simulink model "Consigna5_2_1"  (R2024b)
settings: Solver=ode45  StartTime=0.0  StopTime=20  RelTol=1e-3
values from neighbouring files (symbols this model uses):
  A_corrientes = [0 1; -omega_n_corrientes^2 -2*omega_n_corrientes]    [parametros.m]
  A_inversor = [0 1; -omega_n_inversor^2 -2*omega_n_inversor]    [parametros.m]
  A_posicion = [0 1; -omega_n_posicion^2 -2*omega_n_posicion]    [parametros.m]
  A_temp = -1/20    (= -0.05)    [parametros.m]
  alpha_cu = 3.9 *10^-3    (= 0.0039)    [parametros.m]
  B_corrientes = [0; omega_n_corrientes^2]    [parametros.m]
  b_eq = b_m + (1/r^2) * b_l    (= 2.19444444444e-05)    [parametros.m]
  B_inversor = [0; omega_n_inversor^2]    [parametros.m]
  b_l = 0.1    [parametros.m]
  b_m = 1.5 * 10^-5    (= 1.5e-05)    [parametros.m]
  B_posicion = [0; omega_n_posicion^2]    [parametros.m]
  B_temp = 1/20    (= 0.05)    [parametros.m]
  ba = J_eq*n*omega_pos    (= 0.0916527777778)    [parametros.m]
  C_corrientes = [1 0]    [parametros.m]
  C_inversor = [1 0]    [parametros.m]
  C_posicion = [1 0]    [parametros.m]
  C_temp = 1    [parametros.m]
  C_ts = 0.818    [parametros.m]
  g = 9.80665    [parametros.m]
  J_l = (m*l_cm^2 + J_cm) + (m_l * l_l^2)    (= 0.4583)    [parametros.m]
  J_m = 1.4 * 10^-5    (= 1.4e-05)    [parametros.m]
  K_e_int = 3200 ^3    (= 32768000000)    [parametros.m]
  K_e_omega = 3*3200^2    (= 30720000)    [parametros.m]
  K_e_theta = 9600    [parametros.m]
  k_l = m * l_cm + m_l* l_l    (= 1)    [parametros.m]
  Ksa = J_eq*n*(omega_pos^2)    (= 73.3222222222)    [parametros.m]
  Ksia = J_eq*(omega_pos^3)    (= 23463.1111111)    [parametros.m]
  L_d = 6.6 * 10^-3    (= 0.0066)    [parametros.m]
  L_ls = 0.8 * 10^-3    (= 0.0008)    [parametros.m]
  L_q = 5.8 * 10^-3    (= 0.0058)    [parametros.m]
  lambda_m = 0.016    [parametros.m]
  P_p = 3    [parametros.m]
  r = 120    [parametros.m]
  R_s_40 = 1.02    [parametros.m]
  R_ts_amb = 146.7    [parametros.m]
  T_sample = 1/f_sample    (= 4.53514739229e-05)    [parametros.m]
  Temp_s_ref = 20    [parametros.m]
  tm = X(1)    [parametros.m]
  tr = X(2)    [parametros.m]
  w2 = 188.49556    [parametros.m]
  x0_corrientes = [0;0]    [parametros.m]
  x0_inversor = [0;0]    [parametros.m]
  x0_posicion = [0; 0]    [parametros.m]
  x0_temp = 20    [parametros.m]
libraries: simulink x14, dspsigops x6
(part 3 of 4)

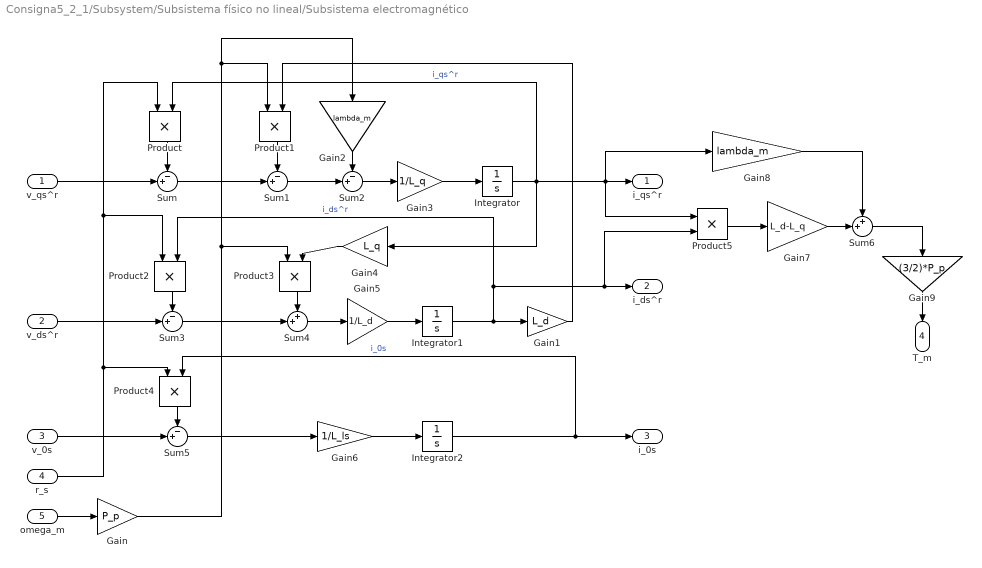
== system Consigna5_2_1/Subsystem/Subsistema físico no lineal/Subsistema electromagnético ==
  v_qs^r : Inport
  v_ds^r : Inport  Port=2
  v_0s : Inport  Port=3
  r_s : Inport  Port=4
  omega_m : Inport  Port=5
  Gain : Gain  Gain=P_p
  Gain1 : Gain  Gain=L_d
  Gain2 : Gain  Gain=lambda_m
  Gain3 : Gain  Gain=1/L_q
  Gain4 : Gain  Gain=L_q
  Gain5 : Gain  Gain=1/L_d
  Gain6 : Gain  Gain=1/L_ls
  Gain7 : Gain  Gain=L_d-L_q
  Gain8 : Gain  Gain=lambda_m
  Gain9 : Gain  Gain=(3/2)*P_p
  Integrator : Integrator
  Integrator1 : Integrator
  Integrator2 : Integrator
  Product{,1..5} (6 alike) : Product
  Sum{,1..3,5} (5 alike) : Sum  Inputs=-+|
  Sum4 : Sum  Inputs=++|
  Sum6 : Sum  Inputs=++|
  i_qs^r : Outport
  i_ds^r : Outport  Port=2
  i_0s : Outport  Port=3
  T_m : Outport  Port=4
  wires:
  v_qs^r/1 -> Sum/2
  Product/1 -> Sum/1
  Sum/1 -> Sum1/2
  Integrator/1 -> Gain8/1, Product5/1, i_qs^r/1, Product/2, Gain4/1  "i_qs^r"
  omega_m/1 -> Gain/1
  Gain/1 -> Gain2/1, Product1/1, Product3/1
  Integrator1/1 -> Product2/2, Product5/2, i_ds^r/1, Gain1/1  "i_ds^r"
  Gain1/1 -> Product1/2
  Sum1/1 -> Sum2/2
  Sum2/1 -> Gain3/1
  Gain2/1 -> Sum2/1
  Product1/1 -> Sum1/1
  Gain3/1 -> Integrator/1
  Product2/1 -> Sum3/1
  v_ds^r/1 -> Sum3/2
  Sum3/1 -> Sum4/2
  Product3/1 -> Sum4/1
  Gain4/1 -> Product3/2
  Gain5/1 -> Integrator1/1
  Sum4/1 -> Gain5/1
  Integrator2/1 -> Product4/2, i_0s/1  "i_0s"
  r_s/1 -> Product4/1, Product/1, Product2/1
  Product4/1 -> Sum5/1
  v_0s/1 -> Sum5/2
  Sum5/1 -> Gain6/1
  Gain6/1 -> Integrator2/1
  Product5/1 -> Gain7/1
  Gain7/1 -> Sum6/2
  Gain8/1 -> Sum6/1
  Sum6/1 -> Gain9/1
  Gain9/1 -> T_m/1

== system Consigna5_2_1/Subsystem/Subsistema físico no lineal/Subsistema mecánico completo ==
  T_m : Inport
  T_l : Inport  Port=2
  Gain : Gain  Gain=b_m + b_l / (r^2)
  Gain1 : Gain  Gain=1/r
  Gain2 : Gain  Gain=1/(J_m + J_l / r^2)
  Scope : Scope
  Sum : Sum  Inputs=-+-
  omega_m(0) = 0 : Integrator
  theta_m(0) = pi/4 : Integrator  InitialCondition=pi/4
  theta_m(t) : Outport
  omega_m(t) : Outport  Port=2
  wires:
  Gain2/1 -> omega_m(0) = 0/1  "domega_m(t)/dt"
  Gain1/1 -> Sum/1
  theta_m(0) = pi/4/1 -> Scope/1, theta_m(t)/1  "theta_m(t)"
  omega_m(0) = 0/1 -> omega_m(t)/1, Gain/1, theta_m(0) = pi/4/1  "omega_m(t)"
  Sum/1 -> Gain2/1
  Gain/1 -> Sum/3
  T_l/1 -> Gain1/1
  T_m/1 -> Sum/2

== system Consigna5_2_1/Subsystem/Subsistema físico no lineal/Subsistema térmico ==
  i_qs^r : Inport
  i_ds^r : Inport  Port=2
  i_0s^r : Inport  Port=3
  Tº_amb : Inport  Port=4
  Constant : Constant  Value=Temp_s_ref
  Constant1 : Constant
  Gain : Gain  Gain=1/C_ts
  Gain1 : Gain  Gain=3/2
  Gain2 : Gain  Gain=1/R_ts_amb
  Gain3 : Gain  Gain=alpha_cu
  Gain4 : Gain  Gain=R_s_40
  Gain5 : Gain  Gain=2
  Integrator : Integrator  InitialCondition=20
  Product : Product
  Square : Math  Operator=square
  Square1 : Math  Operator=square
  Square2 : Math  Operator=square
  Sum : Sum  Inputs=+++
  Sum1 : Sum  Inputs=-|+
  Sum2 : Sum  Inputs=|+-
  Sum3 : Sum  Inputs=|+-
  Sum4 : Sum  Inputs=|++
  r_s : Outport
  T_s : Outport  Port=2
  wires:
  i_qs^r/1 -> Square/1
  i_ds^r/1 -> Square1/1
  i_0s^r/1 -> Square2/1
  Gain/1 -> Integrator/1
  Square/1 -> Sum/1
  Square1/1 -> Sum/2
  Sum/1 -> Product/1
  Product/1 -> Gain1/1
  Tº_amb/1 -> Sum1/1
  Integrator/1 -> T_s/1, Sum3/1, Sum1/2
  Sum1/1 -> Gain2/1
  Gain1/1 -> Sum2/1
  Gain2/1 -> Sum2/2
  Sum2/1 -> Gain/1
  Constant/1 -> Sum3/2
  Sum3/1 -> Gain3/1
  Gain3/1 -> Sum4/1
  Constant1/1 -> Sum4/2
  Sum4/1 -> Gain4/1
  Gain4/1 -> Product/2, r_s/1
  Square2/1 -> Gain5/1
  Gain5/1 -> Sum/3

== system Consigna5_2_1/Subsystem/Subsystem2/Desacoples Fisicos ==
  v_qs* : Inport
  v_ds* : Inport  Port=2
  v_0s* : Inport  Port=3
  i_qs : Inport  Port=4
  i_ds : Inport  Port=5
  i_0s : Inport  Port=6
  omega_m : Inport  Port=7
  R_s : Inport  Port=8
  Constant : Constant  Value=lambda_m
  Gain : Gain  Gain=P_p
  Gain1 : Gain  Gain=L_d
  Gain2 : Gain  Gain=L_q*P_p
  Product{,1..4} (5 alike) : Product
  Sum : Sum  Inputs=|++
  Sum1 : Sum  Inputs=|++
  Sum2 : Sum  Inputs=++|
  Sum3 : Sum  Inputs=+-|
  Sum4 : Sum  Inputs=|++
  Sum5 : Sum  Inputs=++|
  v_qs*' : Outport
  v_ds*' : Outport  Port=2
  v_0s*' : Outport  Port=3
  wires:
  Gain/1 -> Product1/2
  Product2/1 -> Sum3/1
  Sum2/1 -> Product1/1
  Sum1/1 -> v_qs*'/1
  i_ds/1 -> Gain1/1, Product2/2
  i_qs/1 -> Gain2/1, Product/2
  v_qs*/1 -> Sum/1
  v_0s*/1 -> Sum5/2
  v_ds*/1 -> Sum4/1
  Sum/1 -> Sum1/1
  R_s/1 -> Product2/1, Product4/1, Product/1
  Sum4/1 -> v_ds*'/1
  Gain2/1 -> Product3/1
  Sum5/1 -> v_0s*'/1
  Product3/1 -> Sum3/2
  omega_m/1 -> Product3/2, Gain/1
  Constant/1 -> Sum2/1
  Product/1 -> Sum/2
  Gain1/1 -> Sum2/2
  Sum3/1 -> Sum4/2
  Product4/1 -> Sum5/1
  i_0s/1 -> Product4/2
  Product1/1 -> Sum1/2

== system Consigna5_2_1/Subsystem/Subsystem2/Lazo de Torque ==
  Tm* : Inport
  omega_m : Inport  Port=2
  ids : Inport  Port=3
  Constant : Constant  Value=lambda_m
  Constant1 : Constant  Value=g
  Divide : Product  Inputs=*/
  Integrator : Integrator  InitialCondition=pi/4
  Ld-Lq : Constant  Value=L_d-L_q
  Multiply : Gain  Gain=b_eq
  Multiply1 : Gain  Gain=1/r
  Multiply2 : Gain  Gain=k_l
  Multiply3 : Gain  Gain=1/r
  Multiply5 : Gain  Gain=P_p
  Multiply6 : Gain  Gain=3/2
  Product : Product
  Product1 : Product
  Sin : Trigonometry
  Sum1 : Sum  Inputs=|++
  Sum2 : Sum  Inputs=|+++
  iqs* : Outport
  wires:
  Constant/1 -> Sum1/2
  Ld-Lq/1 -> Product1/2
  omega_m/1 -> Integrator/1, Multiply/1
  Tm*/1 -> Sum2/1
  ids/1 -> Product1/1
  Multiply3/1 -> Product/1
  Product/1 -> Sum2/3
  Multiply6/1 -> Divide/2
  Multiply2/1 -> Multiply3/1
  Integrator/1 -> Multiply1/1
  Multiply1/1 -> Sin/1
  Multiply/1 -> Sum2/2
  Sum2/1 -> Divide/1
  Multiply5/1 -> Multiply6/1
  Divide/1 -> iqs*/1
  Sum1/1 -> Multiply5/1
  Sin/1 -> Multiply2/1
  Constant1/1 -> Product/2
  Product1/1 -> Sum1/1

== system Consigna5_2_1/Subsystem/Subsystem2/Modulador de corriente ==
  I_qs* : Inport
  I_ds* : Inport  Port=2
  I_0s* : Inport  Port=3
  i_qs : Inport  Port=4
  i_ds : Inport  Port=5
  i_0s : Inport  Port=6
  Gain : Gain  Gain=5000*L_q
  Gain1 : Gain  Gain=5000*L_d
  Gain2 : Gain  Gain=5000*L_ls
  Sum : Sum  Inputs=+-
  Sum1 : Sum  Inputs=+-
  Sum2 : Sum  Inputs=+-
  v_qs* : Outport
  v_ds* : Outport  Port=2
  v_0s* : Outport  Port=3
  wires:
  Sum2/1 -> Gain2/1
  Sum1/1 -> Gain1/1
  Sum/1 -> Gain/1
  I_qs*/1 -> Sum/1
  i_qs/1 -> Sum/2
  I_ds*/1 -> Sum1/1
  i_ds/1 -> Sum1/2
  I_0s*/1 -> Sum2/1
  i_0s/1 -> Sum2/2
  Gain/1 -> v_qs*/1
  Gain2/1 -> v_0s*/1
  Gain1/1 -> v_ds*/1

== system Consigna5_2_1/Subsystem1/MODULADOR DE TORQUE1/Calculo rs ==
  Ts : Inport
  Constant : Constant
  Constant1 : Constant  Value=Temp_s_ref
  Gain : Gain  Gain=alpha_cu
  Gain1 : Gain  Gain=R_s_40
  Sum : Sum  Inputs=|++
  Sum1 : Sum  Inputs=|-+
  r_s : Outport
  wires:
  Constant/1 -> Sum/1
  Gain/1 -> Sum/2
  Ts/1 -> Sum1/2
  Constant1/1 -> Sum1/1
  Sum1/1 -> Gain/1
  Sum/1 -> Gain1/1
  Gain1/1 -> r_s/1

== system Consigna5_2_1/Subsystem1/MODULADOR DE TORQUE1/Desacoples Fisicos ==
  v_qs* : Inport
  v_ds* : Inport  Port=2
  v_0s* : Inport  Port=3
  i_qs : Inport  Port=4
  i_ds : Inport  Port=5
  i_0s : Inport  Port=6
  omega_m : Inport  Port=7
  R_s : Inport  Port=8
  Constant : Constant  Value=lambda_m
  Gain : Gain  Gain=P_p
  Gain1 : Gain  Gain=L_d
  Gain2 : Gain  Gain=L_q*P_p
  Product{,1..4} (5 alike) : Product
  Sum : Sum  Inputs=|++
  Sum1 : Sum  Inputs=|++
  Sum2 : Sum  Inputs=++|
  Sum3 : Sum  Inputs=+-|
  Sum4 : Sum  Inputs=|++
  Sum5 : Sum  Inputs=++|
  v_qs*' : Outport
  v_ds*' : Outport  Port=2
  v_0s*' : Outport  Port=3
  wires:
  Gain/1 -> Product1/2
  Product2/1 -> Sum3/1
  Sum2/1 -> Product1/1
  Sum1/1 -> v_qs*'/1
  i_ds/1 -> Gain1/1, Product2/2
  i_qs/1 -> Gain2/1, Product/2
  v_qs*/1 -> Sum/1
  v_0s*/1 -> Sum5/2
  v_ds*/1 -> Sum4/1
  Sum/1 -> Sum1/1
  R_s/1 -> Product2/1, Product4/1, Product/1
  Sum4/1 -> v_ds*'/1
  Gain2/1 -> Product3/1
  Sum5/1 -> v_0s*'/1
  Product3/1 -> Sum3/2
  omega_m/1 -> Product3/2, Gain/1
  Constant/1 -> Sum2/1
  Product/1 -> Sum/2
  Gain1/1 -> Sum2/2
  Sum3/1 -> Sum4/2
  Product4/1 -> Sum5/1
  i_0s/1 -> Product4/2
  Product1/1 -> Sum1/2

== system Consigna5_2_1/Subsystem1/MODULADOR DE TORQUE1/Lazo de Torque ==
  Tm* : Inport
  omega_m : Inport  Port=2
  ids : Inport  Port=3
  Constant : Constant  Value=lambda_m
  Constant1 : Constant  Value=g
  Divide : Product  Inputs=*/
  Integrator : Integrator  InitialCondition=pi/4
  Ld-Lq : Constant  Value=L_d-L_q
  Multiply : Gain  Gain=b_eq
  Multiply1 : Gain  Gain=1/r
  Multiply2 : Gain  Gain=k_l
  Multiply3 : Gain  Gain=1/r
  Multiply5 : Gain  Gain=P_p
  Multiply6 : Gain  Gain=3/2
  Product : Product
  Product1 : Product
  Sin : Trigonometry
  Sum1 : Sum  Inputs=|++
  Sum2 : Sum  Inputs=|+++
  iqs* : Outport
  wires:
  Constant/1 -> Sum1/2
  Ld-Lq/1 -> Product1/2
  omega_m/1 -> Integrator/1, Multiply/1
  Tm*/1 -> Sum2/1
  ids/1 -> Product1/1
  Multiply3/1 -> Product/1
  Product/1 -> Sum2/3
  Multiply6/1 -> Divide/2
  Multiply2/1 -> Multiply3/1
  Integrator/1 -> Multiply1/1
  Multiply1/1 -> Sin/1
  Multiply/1 -> Sum2/2
  Sum2/1 -> Divide/1
  Multiply5/1 -> Multiply6/1
  Divide/1 -> iqs*/1
  Sum1/1 -> Multiply5/1
  Sin/1 -> Multiply2/1
  Constant1/1 -> Product/2
  Product1/1 -> Sum1/1

== system Consigna5_2_1/Subsystem1/MODULADOR DE TORQUE1/Modulador de corriente ==
  I_qs* : Inport
  I_ds* : Inport  Port=2
  I_0s* : Inport  Port=3
  i_qs : Inport  Port=4
  i_ds : Inport  Port=5
  i_0s : Inport  Port=6
  Gain : Gain  Gain=5000*L_q
  Gain1 : Gain  Gain=5000*L_d
  Gain2 : Gain  Gain=5000*L_ls
  Sum : Sum  Inputs=+-
  Sum1 : Sum  Inputs=+-
  Sum2 : Sum  Inputs=+-
  v_qs* : Outport
  v_ds* : Outport  Port=2
  v_0s* : Outport  Port=3
  wires:
  Sum2/1 -> Gain2/1
  Sum1/1 -> Gain1/1
  Sum/1 -> Gain/1
  I_qs*/1 -> Sum/1
  i_qs/1 -> Sum/2
  I_ds*/1 -> Sum1/1
  i_ds/1 -> Sum1/2
  I_0s*/1 -> Sum2/1
  i_0s/1 -> Sum2/2
  Gain/1 -> v_qs*/1
  Gain2/1 -> v_0s*/1
  Gain1/1 -> v_ds*/1

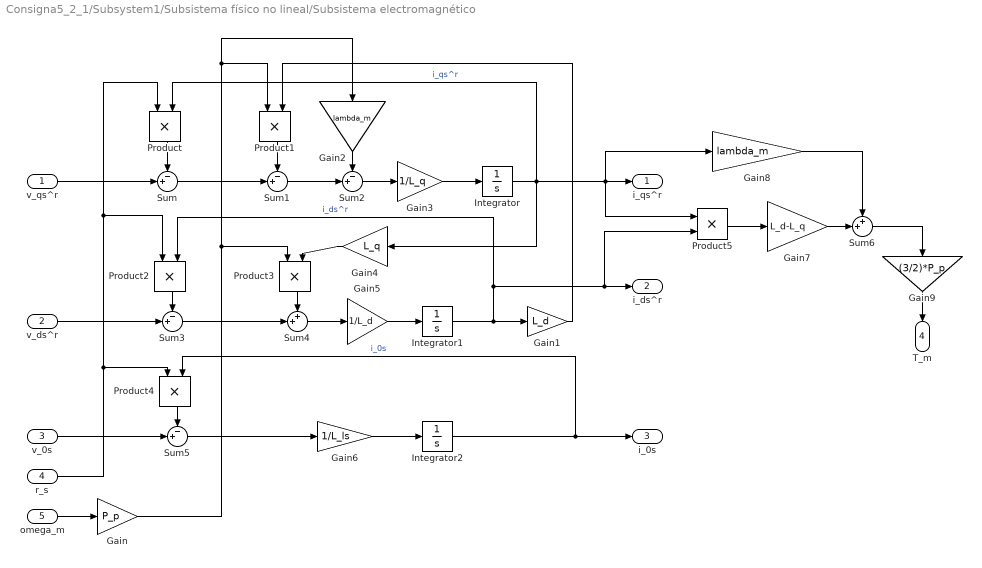
== system Consigna5_2_1/Subsystem1/Subsistema físico no lineal/Subsistema electromagnético ==
  v_qs^r : Inport
  v_ds^r : Inport  Port=2
  v_0s : Inport  Port=3
  r_s : Inport  Port=4
  omega_m : Inport  Port=5
  Gain : Gain  Gain=P_p
  Gain1 : Gain  Gain=L_d
  Gain2 : Gain  Gain=lambda_m
  Gain3 : Gain  Gain=1/L_q
  Gain4 : Gain  Gain=L_q
  Gain5 : Gain  Gain=1/L_d
  Gain6 : Gain  Gain=1/L_ls
  Gain7 : Gain  Gain=L_d-L_q
  Gain8 : Gain  Gain=lambda_m
  Gain9 : Gain  Gain=(3/2)*P_p
  Integrator : Integrator
  Integrator1 : Integrator
  Integrator2 : Integrator
  Product{,1..5} (6 alike) : Product
  Sum{,1..3,5} (5 alike) : Sum  Inputs=-+|
  Sum4 : Sum  Inputs=++|
  Sum6 : Sum  Inputs=++|
  i_qs^r : Outport
  i_ds^r : Outport  Port=2
  i_0s : Outport  Port=3
  T_m : Outport  Port=4
  wires:
  v_qs^r/1 -> Sum/2
  Product/1 -> Sum/1
  Sum/1 -> Sum1/2
  Integrator/1 -> Gain8/1, Product5/1, i_qs^r/1, Product/2, Gain4/1  "i_qs^r"
  omega_m/1 -> Gain/1
  Gain/1 -> Gain2/1, Product1/1, Product3/1
  Integrator1/1 -> Product2/2, Product5/2, i_ds^r/1, Gain1/1  "i_ds^r"
  Gain1/1 -> Product1/2
  Sum1/1 -> Sum2/2
  Sum2/1 -> Gain3/1
  Gain2/1 -> Sum2/1
  Product1/1 -> Sum1/1
  Gain3/1 -> Integrator/1
  Product2/1 -> Sum3/1
  v_ds^r/1 -> Sum3/2
  Sum3/1 -> Sum4/2
  Product3/1 -> Sum4/1
  Gain4/1 -> Product3/2
  Gain5/1 -> Integrator1/1
  Sum4/1 -> Gain5/1
  Integrator2/1 -> Product4/2, i_0s/1  "i_0s"
  r_s/1 -> Product4/1, Product/1, Product2/1
  Product4/1 -> Sum5/1
  v_0s/1 -> Sum5/2
  Sum5/1 -> Gain6/1
  Gain6/1 -> Integrator2/1
  Product5/1 -> Gain7/1
  Gain7/1 -> Sum6/2
  Gain8/1 -> Sum6/1
  Sum6/1 -> Gain9/1
  Gain9/1 -> T_m/1

== system Consigna5_2_1/Subsystem1/Subsistema físico no lineal/Subsistema mecánico completo ==
  T_m : Inport
  T_l : Inport  Port=2
  Gain : Gain  Gain=b_m + b_l / (r^2)
  Gain1 : Gain  Gain=1/r
  Gain2 : Gain  Gain=1/(J_m + J_l / r^2)
  Sum : Sum  Inputs=-+-
  omega_m(0) = 0 : Integrator
  theta_m(0) = 0 : Integrator
  theta_m(t) : Outport
  omega_m(t) : Outport  Port=2
  wires:
  Gain2/1 -> omega_m(0) = 0/1  "domega_m(t)/dt"
  Gain1/1 -> Sum/1
  theta_m(0) = 0/1 -> theta_m(t)/1  "theta_m(t)"
  omega_m(0) = 0/1 -> omega_m(t)/1, Gain/1, theta_m(0) = 0/1  "omega_m(t)"
  Sum/1 -> Gain2/1
  Gain/1 -> Sum/3
  T_l/1 -> Gain1/1
  T_m/1 -> Sum/2

== system Consigna5_2_1/Subsystem1/Subsistema físico no lineal/Subsistema térmico ==
  i_qs^r : Inport
  i_ds^r : Inport  Port=2
  i_0s^r : Inport  Port=3
  Tº_amb : Inport  Port=4
  Constant : Constant  Value=Temp_s_ref
  Constant1 : Constant
  Gain : Gain  Gain=1/C_ts
  Gain1 : Gain  Gain=3/2
  Gain2 : Gain  Gain=1/R_ts_amb
  Gain3 : Gain  Gain=alpha_cu
  Gain4 : Gain  Gain=R_s_40
  Gain5 : Gain  Gain=2
  Integrator : Integrator  InitialCondition=20
  Product : Product
  Square : Math  Operator=square
  Square1 : Math  Operator=square
  Square2 : Math  Operator=square
  Sum : Sum  Inputs=+++
  Sum1 : Sum  Inputs=-|+
  Sum2 : Sum  Inputs=|+-
  Sum3 : Sum  Inputs=|+-
  Sum4 : Sum  Inputs=|++
  r_s : Outport
  T_s : Outport  Port=2
  wires:
  i_qs^r/1 -> Square/1
  i_ds^r/1 -> Square1/1
  i_0s^r/1 -> Square2/1
  Gain/1 -> Integrator/1
  Square/1 -> Sum/1
  Square1/1 -> Sum/2
  Sum/1 -> Product/1
  Product/1 -> Gain1/1
  Tº_amb/1 -> Sum1/1
  Integrator/1 -> T_s/1, Sum3/1, Sum1/2
  Sum1/1 -> Gain2/1
  Gain1/1 -> Sum2/1
  Gain2/1 -> Sum2/2
  Sum2/1 -> Gain/1
  Constant/1 -> Sum3/2
  Sum3/1 -> Gain3/1
  Gain3/1 -> Sum4/1
  Constant1/1 -> Sum4/2
  Sum4/1 -> Gain4/1
  Gain4/1 -> Product/2, r_s/1
  Square2/1 -> Gain5/1
  Gain5/1 -> Sum/3

== system Consigna5_2_1/Subsystem2/MODULADOR DE TORQUE1/Calculo rs ==
  Ts : Inport
  Constant : Constant
  Constant1 : Constant  Value=Temp_s_ref
  Gain : Gain  Gain=alpha_cu
  Gain1 : Gain  Gain=R_s_40
  Sum : Sum  Inputs=|++
  Sum1 : Sum  Inputs=|-+
  r_s : Outport
  wires:
  Constant/1 -> Sum/1
  Gain/1 -> Sum/2
  Ts/1 -> Sum1/2
  Constant1/1 -> Sum1/1
  Sum1/1 -> Gain/1
  Sum/1 -> Gain1/1
  Gain1/1 -> r_s/1

== system Consigna5_2_1/Subsystem2/MODULADOR DE TORQUE1/Desacoples Fisicos ==
  v_qs* : Inport
  v_ds* : Inport  Port=2
  v_0s* : Inport  Port=3
  i_qs : Inport  Port=4
  i_ds : Inport  Port=5
  i_0s : Inport  Port=6
  omega_m : Inport  Port=7
  R_s : Inport  Port=8
  Constant : Constant  Value=lambda_m
  Gain : Gain  Gain=P_p
  Gain1 : Gain  Gain=L_d
  Gain2 : Gain  Gain=L_q*P_p
  Product{,1..4} (5 alike) : Product
  Sum : Sum  Inputs=|++
  Sum1 : Sum  Inputs=|++
  Sum2 : Sum  Inputs=++|
  Sum3 : Sum  Inputs=+-|
  Sum4 : Sum  Inputs=|++
  Sum5 : Sum  Inputs=++|
  v_qs*' : Outport
  v_ds*' : Outport  Port=2
  v_0s*' : Outport  Port=3
  wires:
  Gain/1 -> Product1/2
  Product2/1 -> Sum3/1
  Sum2/1 -> Product1/1
  Sum1/1 -> v_qs*'/1
  i_ds/1 -> Gain1/1, Product2/2
  i_qs/1 -> Gain2/1, Product/2
  v_qs*/1 -> Sum/1
  v_0s*/1 -> Sum5/2
  v_ds*/1 -> Sum4/1
  Sum/1 -> Sum1/1
  R_s/1 -> Product2/1, Product4/1, Product/1
  Sum4/1 -> v_ds*'/1
  Gain2/1 -> Product3/1
  Sum5/1 -> v_0s*'/1
  Product3/1 -> Sum3/2
  omega_m/1 -> Product3/2, Gain/1
  Constant/1 -> Sum2/1
  Product/1 -> Sum/2
  Gain1/1 -> Sum2/2
  Sum3/1 -> Sum4/2
  Product4/1 -> Sum5/1
  i_0s/1 -> Product4/2
  Product1/1 -> Sum1/2

== system Consigna5_2_1/Subsystem2/MODULADOR DE TORQUE1/Lazo de Torque ==
  Tm* : Inport
  omega_m : Inport  Port=2
  ids : Inport  Port=3
  Constant : Constant  Value=lambda_m
  Constant1 : Constant  Value=g
  Divide : Product  Inputs=*/
  Integrator : Integrator  InitialCondition=pi/4
  Ld-Lq : Constant  Value=L_d-L_q
  Multiply : Gain  Gain=b_eq
  Multiply1 : Gain  Gain=1/r
  Multiply2 : Gain  Gain=k_l
  Multiply3 : Gain  Gain=1/r
  Multiply5 : Gain  Gain=P_p
  Multiply6 : Gain  Gain=3/2
  Product : Product
  Product1 : Product
  Sin : Trigonometry
  Sum1 : Sum  Inputs=|++
  Sum2 : Sum  Inputs=|+++
  iqs* : Outport
  wires:
  Constant/1 -> Sum1/2
  Ld-Lq/1 -> Product1/2
  omega_m/1 -> Integrator/1, Multiply/1
  Tm*/1 -> Sum2/1
  ids/1 -> Product1/1
  Multiply3/1 -> Product/1
  Product/1 -> Sum2/3
  Multiply6/1 -> Divide/2
  Multiply2/1 -> Multiply3/1
  Integrator/1 -> Multiply1/1
  Multiply1/1 -> Sin/1
  Multiply/1 -> Sum2/2
  Sum2/1 -> Divide/1
  Multiply5/1 -> Multiply6/1
  Divide/1 -> iqs*/1
  Sum1/1 -> Multiply5/1
  Sin/1 -> Multiply2/1
  Constant1/1 -> Product/2
  Product1/1 -> Sum1/1

== system Consigna5_2_1/Subsystem2/MODULADOR DE TORQUE1/Modulador de corriente ==
  I_qs* : Inport
  I_ds* : Inport  Port=2
  I_0s* : Inport  Port=3
  i_qs : Inport  Port=4
  i_ds : Inport  Port=5
  i_0s : Inport  Port=6
  Gain : Gain  Gain=5000*L_q
  Gain1 : Gain  Gain=5000*L_d
  Gain2 : Gain  Gain=5000*L_ls
  Sum : Sum  Inputs=+-
  Sum1 : Sum  Inputs=+-
  Sum2 : Sum  Inputs=+-
  v_qs* : Outport
  v_ds* : Outport  Port=2
  v_0s* : Outport  Port=3
  wires:
  Sum2/1 -> Gain2/1
  Sum1/1 -> Gain1/1
  Sum/1 -> Gain/1
  I_qs*/1 -> Sum/1
  i_qs/1 -> Sum/2
  I_ds*/1 -> Sum1/1
  i_ds/1 -> Sum1/2
  I_0s*/1 -> Sum2/1
  i_0s/1 -> Sum2/2
  Gain/1 -> v_qs*/1
  Gain2/1 -> v_0s*/1
  Gain1/1 -> v_ds*/1

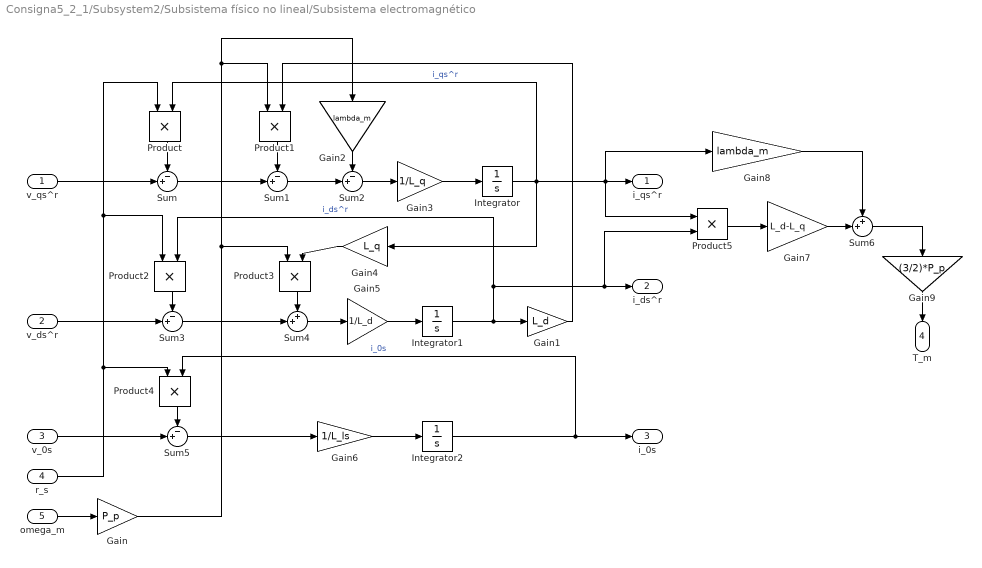
== system Consigna5_2_1/Subsystem2/Subsistema físico no lineal/Subsistema electromagnético ==
  v_qs^r : Inport
  v_ds^r : Inport  Port=2
  v_0s : Inport  Port=3
  r_s : Inport  Port=4
  omega_m : Inport  Port=5
  Gain : Gain  Gain=P_p
  Gain1 : Gain  Gain=L_d
  Gain2 : Gain  Gain=lambda_m
  Gain3 : Gain  Gain=1/L_q
  Gain4 : Gain  Gain=L_q
  Gain5 : Gain  Gain=1/L_d
  Gain6 : Gain  Gain=1/L_ls
  Gain7 : Gain  Gain=L_d-L_q
  Gain8 : Gain  Gain=lambda_m
  Gain9 : Gain  Gain=(3/2)*P_p
  Integrator : Integrator
  Integrator1 : Integrator
  Integrator2 : Integrator
  Product{,1..5} (6 alike) : Product
  Sum{,1..3,5} (5 alike) : Sum  Inputs=-+|
  Sum4 : Sum  Inputs=++|
  Sum6 : Sum  Inputs=++|
  i_qs^r : Outport
  i_ds^r : Outport  Port=2
  i_0s : Outport  Port=3
  T_m : Outport  Port=4
  wires:
  v_qs^r/1 -> Sum/2
  Product/1 -> Sum/1
  Sum/1 -> Sum1/2
  Integrator/1 -> Gain8/1, Product5/1, i_qs^r/1, Product/2, Gain4/1  "i_qs^r"
  omega_m/1 -> Gain/1
  Gain/1 -> Gain2/1, Product1/1, Product3/1
  Integrator1/1 -> Product2/2, Product5/2, i_ds^r/1, Gain1/1  "i_ds^r"
  Gain1/1 -> Product1/2
  Sum1/1 -> Sum2/2
  Sum2/1 -> Gain3/1
  Gain2/1 -> Sum2/1
  Product1/1 -> Sum1/1
  Gain3/1 -> Integrator/1
  Product2/1 -> Sum3/1
  v_ds^r/1 -> Sum3/2
  Sum3/1 -> Sum4/2
  Product3/1 -> Sum4/1
  Gain4/1 -> Product3/2
  Gain5/1 -> Integrator1/1
  Sum4/1 -> Gain5/1
  Integrator2/1 -> Product4/2, i_0s/1  "i_0s"
  r_s/1 -> Product4/1, Product/1, Product2/1
  Product4/1 -> Sum5/1
  v_0s/1 -> Sum5/2
  Sum5/1 -> Gain6/1
  Gain6/1 -> Integrator2/1
  Product5/1 -> Gain7/1
  Gain7/1 -> Sum6/2
  Gain8/1 -> Sum6/1
  Sum6/1 -> Gain9/1
  Gain9/1 -> T_m/1

== system Consigna5_2_1/Subsystem2/Subsistema físico no lineal/Subsistema mecánico completo ==
  T_m : Inport
  T_l : Inport  Port=2
  Gain : Gain  Gain=b_m + b_l / (r^2)
  Gain1 : Gain  Gain=1/r
  Gain2 : Gain  Gain=1/(J_m + J_l / r^2)
  Sum : Sum  Inputs=-+-
  omega_m(0) = 0 : Integrator
  theta_m(0) = 0 : Integrator
  theta_m(t) : Outport
  omega_m(t) : Outport  Port=2
  wires:
  Gain2/1 -> omega_m(0) = 0/1  "domega_m(t)/dt"
  Gain1/1 -> Sum/1
  theta_m(0) = 0/1 -> theta_m(t)/1  "theta_m(t)"
  omega_m(0) = 0/1 -> omega_m(t)/1, Gain/1, theta_m(0) = 0/1  "omega_m(t)"
  Sum/1 -> Gain2/1
  Gain/1 -> Sum/3
  T_l/1 -> Gain1/1
  T_m/1 -> Sum/2

== system Consigna5_2_1/Subsystem2/Subsistema físico no lineal/Subsistema térmico ==
  i_qs^r : Inport
  i_ds^r : Inport  Port=2
  i_0s^r : Inport  Port=3
  Tº_amb : Inport  Port=4
  Constant : Constant  Value=Temp_s_ref
  Constant1 : Constant
  Gain : Gain  Gain=1/C_ts
  Gain1 : Gain  Gain=3/2
  Gain2 : Gain  Gain=1/R_ts_amb
  Gain3 : Gain  Gain=alpha_cu
  Gain4 : Gain  Gain=R_s_40
  Gain5 : Gain  Gain=2
  Integrator : Integrator  InitialCondition=20
  Product : Product
  Square : Math  Operator=square
  Square1 : Math  Operator=square
  Square2 : Math  Operator=square
  Sum : Sum  Inputs=+++
  Sum1 : Sum  Inputs=-|+
  Sum2 : Sum  Inputs=|+-
  Sum3 : Sum  Inputs=|+-
  Sum4 : Sum  Inputs=|++
  r_s : Outport
  T_s : Outport  Port=2
  wires:
  i_qs^r/1 -> Square/1
  i_ds^r/1 -> Square1/1
  i_0s^r/1 -> Square2/1
  Gain/1 -> Integrator/1
  Square/1 -> Sum/1
  Square1/1 -> Sum/2
  Sum/1 -> Product/1
  Product/1 -> Gain1/1
  Tº_amb/1 -> Sum1/1
  Integrator/1 -> T_s/1, Sum3/1, Sum1/2
  Sum1/1 -> Gain2/1
  Gain1/1 -> Sum2/1
  Gain2/1 -> Sum2/2
  Sum2/1 -> Gain/1
  Constant/1 -> Sum3/2
  Sum3/1 -> Gain3/1
  Gain3/1 -> Sum4/1
  Constant1/1 -> Sum4/2
  Sum4/1 -> Gain4/1
  Gain4/1 -> Product/2, r_s/1
  Square2/1 -> Gain5/1
  Gain5/1 -> Sum/3

== system Consigna5_2_1/Subsystem3/MODULADOR DE TORQUE1/Calculo rs ==
  Ts : Inport
  Constant : Constant
  Constant1 : Constant  Value=Temp_s_ref
  Gain : Gain  Gain=alpha_cu
  Gain1 : Gain  Gain=R_s_40
  Sum : Sum  Inputs=|++
  Sum1 : Sum  Inputs=|-+
  r_s : Outport
  wires:
  Constant/1 -> Sum/1
  Gain/1 -> Sum/2
  Ts/1 -> Sum1/2
  Constant1/1 -> Sum1/1
  Sum1/1 -> Gain/1
  Sum/1 -> Gain1/1
  Gain1/1 -> r_s/1

== system Consigna5_2_1/Subsystem3/MODULADOR DE TORQUE1/Desacoples Fisicos ==
  v_qs* : Inport
  v_ds* : Inport  Port=2
  v_0s* : Inport  Port=3
  i_qs : Inport  Port=4
  i_ds : Inport  Port=5
  i_0s : Inport  Port=6
  omega_m : Inport  Port=7
  R_s : Inport  Port=8
  Constant : Constant  Value=lambda_m
  Gain : Gain  Gain=P_p
  Gain1 : Gain  Gain=L_d
  Gain2 : Gain  Gain=L_q*P_p
  Product{,1..4} (5 alike) : Product
  Sum : Sum  Inputs=|++
  Sum1 : Sum  Inputs=|++
  Sum2 : Sum  Inputs=++|
  Sum3 : Sum  Inputs=+-|
  Sum4 : Sum  Inputs=|++
  Sum5 : Sum  Inputs=++|
  v_qs*' : Outport
  v_ds*' : Outport  Port=2
  v_0s*' : Outport  Port=3
  wires:
  Gain/1 -> Product1/2
  Product2/1 -> Sum3/1
  Sum2/1 -> Product1/1
  Sum1/1 -> v_qs*'/1
  i_ds/1 -> Gain1/1, Product2/2
  i_qs/1 -> Gain2/1, Product/2
  v_qs*/1 -> Sum/1
  v_0s*/1 -> Sum5/2
  v_ds*/1 -> Sum4/1
  Sum/1 -> Sum1/1
  R_s/1 -> Product2/1, Product4/1, Product/1
  Sum4/1 -> v_ds*'/1
  Gain2/1 -> Product3/1
  Sum5/1 -> v_0s*'/1
  Product3/1 -> Sum3/2
  omega_m/1 -> Product3/2, Gain/1
  Constant/1 -> Sum2/1
  Product/1 -> Sum/2
  Gain1/1 -> Sum2/2
  Sum3/1 -> Sum4/2
  Product4/1 -> Sum5/1
  i_0s/1 -> Product4/2
  Product1/1 -> Sum1/2

== system Consigna5_2_1/Subsystem3/MODULADOR DE TORQUE1/Lazo de Torque ==
  Tm* : Inport
  omega_m : Inport  Port=2
  ids : Inport  Port=3
  Constant : Constant  Value=lambda_m
  Constant1 : Constant  Value=g
  Divide : Product  Inputs=*/
  Integrator : Integrator  InitialCondition=pi/4
  Ld-Lq : Constant  Value=L_d-L_q
  Multiply : Gain  Gain=b_eq
  Multiply1 : Gain  Gain=1/r
  Multiply2 : Gain  Gain=k_l
  Multiply3 : Gain  Gain=1/r
  Multiply5 : Gain  Gain=P_p
  Multiply6 : Gain  Gain=3/2
  Product : Product
  Product1 : Product
  Sin : Trigonometry
  Sum1 : Sum  Inputs=|++
  Sum2 : Sum  Inputs=|+++
  iqs* : Outport
  wires:
  Constant/1 -> Sum1/2
  Ld-Lq/1 -> Product1/2
  omega_m/1 -> Integrator/1, Multiply/1
  Tm*/1 -> Sum2/1
  ids/1 -> Product1/1
  Multiply3/1 -> Product/1
  Product/1 -> Sum2/3
  Multiply6/1 -> Divide/2
  Multiply2/1 -> Multiply3/1
  Integrator/1 -> Multiply1/1
  Multiply1/1 -> Sin/1
  Multiply/1 -> Sum2/2
  Sum2/1 -> Divide/1
  Multiply5/1 -> Multiply6/1
  Divide/1 -> iqs*/1
  Sum1/1 -> Multiply5/1
  Sin/1 -> Multiply2/1
  Constant1/1 -> Product/2
  Product1/1 -> Sum1/1

== system Consigna5_2_1/Subsystem3/MODULADOR DE TORQUE1/Modulador de corriente ==
  I_qs* : Inport
  I_ds* : Inport  Port=2
  I_0s* : Inport  Port=3
  i_qs : Inport  Port=4
  i_ds : Inport  Port=5
  i_0s : Inport  Port=6
  Gain : Gain  Gain=5000*L_q
  Gain1 : Gain  Gain=5000*L_d
  Gain2 : Gain  Gain=5000*L_ls
  Sum : Sum  Inputs=+-
  Sum1 : Sum  Inputs=+-
  Sum2 : Sum  Inputs=+-
  v_qs* : Outport
  v_ds* : Outport  Port=2
  v_0s* : Outport  Port=3
  wires:
  Sum2/1 -> Gain2/1
  Sum1/1 -> Gain1/1
  Sum/1 -> Gain/1
  I_qs*/1 -> Sum/1
  i_qs/1 -> Sum/2
  I_ds*/1 -> Sum1/1
  i_ds/1 -> Sum1/2
  I_0s*/1 -> Sum2/1
  i_0s/1 -> Sum2/2
  Gain/1 -> v_qs*/1
  Gain2/1 -> v_0s*/1
  Gain1/1 -> v_ds*/1

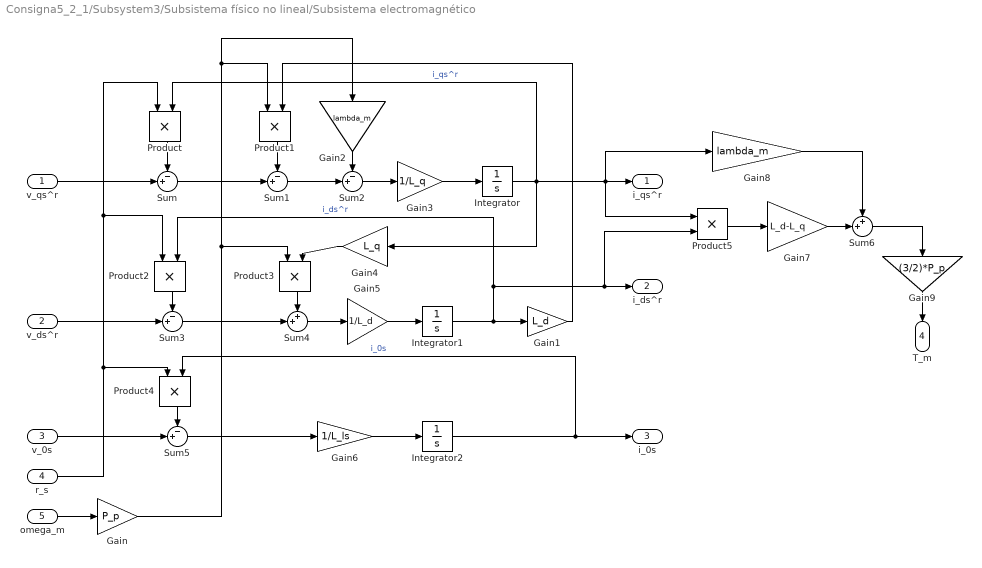
== system Consigna5_2_1/Subsystem3/Subsistema físico no lineal/Subsistema electromagnético ==
  v_qs^r : Inport
  v_ds^r : Inport  Port=2
  v_0s : Inport  Port=3
  r_s : Inport  Port=4
  omega_m : Inport  Port=5
  Gain : Gain  Gain=P_p
  Gain1 : Gain  Gain=L_d
  Gain2 : Gain  Gain=lambda_m
  Gain3 : Gain  Gain=1/L_q
  Gain4 : Gain  Gain=L_q
  Gain5 : Gain  Gain=1/L_d
  Gain6 : Gain  Gain=1/L_ls
  Gain7 : Gain  Gain=L_d-L_q
  Gain8 : Gain  Gain=lambda_m
  Gain9 : Gain  Gain=(3/2)*P_p
  Integrator : Integrator
  Integrator1 : Integrator
  Integrator2 : Integrator
  Product{,1..5} (6 alike) : Product
  Sum{,1..3,5} (5 alike) : Sum  Inputs=-+|
  Sum4 : Sum  Inputs=++|
  Sum6 : Sum  Inputs=++|
  i_qs^r : Outport
  i_ds^r : Outport  Port=2
  i_0s : Outport  Port=3
  T_m : Outport  Port=4
  wires:
  v_qs^r/1 -> Sum/2
  Product/1 -> Sum/1
  Sum/1 -> Sum1/2
  Integrator/1 -> Gain8/1, Product5/1, i_qs^r/1, Product/2, Gain4/1  "i_qs^r"
  omega_m/1 -> Gain/1
  Gain/1 -> Gain2/1, Product1/1, Product3/1
  Integrator1/1 -> Product2/2, Product5/2, i_ds^r/1, Gain1/1  "i_ds^r"
  Gain1/1 -> Product1/2
  Sum1/1 -> Sum2/2
  Sum2/1 -> Gain3/1
  Gain2/1 -> Sum2/1
  Product1/1 -> Sum1/1
  Gain3/1 -> Integrator/1
  Product2/1 -> Sum3/1
  v_ds^r/1 -> Sum3/2
  Sum3/1 -> Sum4/2
  Product3/1 -> Sum4/1
  Gain4/1 -> Product3/2
  Gain5/1 -> Integrator1/1
  Sum4/1 -> Gain5/1
  Integrator2/1 -> Product4/2, i_0s/1  "i_0s"
  r_s/1 -> Product4/1, Product/1, Product2/1
  Product4/1 -> Sum5/1
  v_0s/1 -> Sum5/2
  Sum5/1 -> Gain6/1
  Gain6/1 -> Integrator2/1
  Product5/1 -> Gain7/1
  Gain7/1 -> Sum6/2
  Gain8/1 -> Sum6/1
  Sum6/1 -> Gain9/1
  Gain9/1 -> T_m/1

== system Consigna5_2_1/Subsystem3/Subsistema físico no lineal/Subsistema mecánico completo ==
  T_m : Inport
  T_l : Inport  Port=2
  Gain : Gain  Gain=b_m + b_l / (r^2)
  Gain1 : Gain  Gain=1/r
  Gain2 : Gain  Gain=1/(J_m + J_l / r^2)
  Sum : Sum  Inputs=-+-
  omega_m(0) = 0 : Integrator
  theta_m(0) = 0 : Integrator
  theta_m(t) : Outport
  omega_m(t) : Outport  Port=2
  wires:
  Gain2/1 -> omega_m(0) = 0/1  "domega_m(t)/dt"
  Gain1/1 -> Sum/1
  theta_m(0) = 0/1 -> theta_m(t)/1  "theta_m(t)"
  omega_m(0) = 0/1 -> omega_m(t)/1, Gain/1, theta_m(0) = 0/1  "omega_m(t)"
  Sum/1 -> Gain2/1
  Gain/1 -> Sum/3
  T_l/1 -> Gain1/1
  T_m/1 -> Sum/2

== system Consigna5_2_1/Subsystem3/Subsistema físico no lineal/Subsistema térmico ==
  i_qs^r : Inport
  i_ds^r : Inport  Port=2
  i_0s^r : Inport  Port=3
  Tº_amb : Inport  Port=4
  Constant : Constant  Value=Temp_s_ref
  Constant1 : Constant
  Gain : Gain  Gain=1/C_ts
  Gain1 : Gain  Gain=3/2
  Gain2 : Gain  Gain=1/R_ts_amb
  Gain3 : Gain  Gain=alpha_cu
  Gain4 : Gain  Gain=R_s_40
  Gain5 : Gain  Gain=2
  Integrator : Integrator  InitialCondition=20
  Product : Product
  Square : Math  Operator=square
  Square1 : Math  Operator=square
  Square2 : Math  Operator=square
  Sum : Sum  Inputs=+++
  Sum1 : Sum  Inputs=-|+
  Sum2 : Sum  Inputs=|+-
  Sum3 : Sum  Inputs=|+-
  Sum4 : Sum  Inputs=|++
  r_s : Outport
  T_s : Outport  Port=2
  wires:
  i_qs^r/1 -> Square/1
  i_ds^r/1 -> Square1/1
  i_0s^r/1 -> Square2/1
  Gain/1 -> Integrator/1
  Square/1 -> Sum/1
  Square1/1 -> Sum/2
  Sum/1 -> Product/1
  Product/1 -> Gain1/1
  Tº_amb/1 -> Sum1/1
  Integrator/1 -> T_s/1, Sum3/1, Sum1/2
  Sum1/1 -> Gain2/1
  Gain1/1 -> Sum2/1
  Gain2/1 -> Sum2/2
  Sum2/1 -> Gain/1
  Constant/1 -> Sum3/2
  Sum3/1 -> Gain3/1
  Gain3/1 -> Sum4/1
  Constant1/1 -> Sum4/2
  Sum4/1 -> Gain4/1
  Gain4/1 -> Product/2, r_s/1
  Square2/1 -> Gain5/1
  Gain5/1 -> Sum/3

== system Consigna5_2_1/Subsystem4/MODULADOR DE TORQUE1/Calculo rs ==
  Ts : Inport
  Constant : Constant
  Constant1 : Constant  Value=Temp_s_ref
  Gain : Gain  Gain=alpha_cu
  Gain1 : Gain  Gain=R_s_40
  Sum : Sum  Inputs=|++
  Sum1 : Sum  Inputs=|-+
  r_s : Outport
  wires:
  Constant/1 -> Sum/1
  Gain/1 -> Sum/2
  Ts/1 -> Sum1/2
  Constant1/1 -> Sum1/1
  Sum1/1 -> Gain/1
  Sum/1 -> Gain1/1
  Gain1/1 -> r_s/1

== system Consigna5_2_1/Subsystem4/MODULADOR DE TORQUE1/Desacoples Fisicos ==
  v_qs* : Inport
  v_ds* : Inport  Port=2
  v_0s* : Inport  Port=3
  i_qs : Inport  Port=4
  i_ds : Inport  Port=5
  i_0s : Inport  Port=6
  omega_m : Inport  Port=7
  R_s : Inport  Port=8
  Constant : Constant  Value=lambda_m
  Gain : Gain  Gain=P_p
  Gain1 : Gain  Gain=L_d
  Gain2 : Gain  Gain=L_q*P_p
  Product{,1..4} (5 alike) : Product
  Sum : Sum  Inputs=|++
  Sum1 : Sum  Inputs=|++
  Sum2 : Sum  Inputs=++|
  Sum3 : Sum  Inputs=+-|
  Sum4 : Sum  Inputs=|++
  Sum5 : Sum  Inputs=++|
  v_qs*' : Outport
  v_ds*' : Outport  Port=2
  v_0s*' : Outport  Port=3
  wires:
  Gain/1 -> Product1/2
  Product2/1 -> Sum3/1
  Sum2/1 -> Product1/1
  Sum1/1 -> v_qs*'/1
  i_ds/1 -> Gain1/1, Product2/2
  i_qs/1 -> Gain2/1, Product/2
  v_qs*/1 -> Sum/1
  v_0s*/1 -> Sum5/2
  v_ds*/1 -> Sum4/1
  Sum/1 -> Sum1/1
  R_s/1 -> Product2/1, Product4/1, Product/1
  Sum4/1 -> v_ds*'/1
  Gain2/1 -> Product3/1
  Sum5/1 -> v_0s*'/1
  Product3/1 -> Sum3/2
  omega_m/1 -> Product3/2, Gain/1
  Constant/1 -> Sum2/1
  Product/1 -> Sum/2
  Gain1/1 -> Sum2/2
  Sum3/1 -> Sum4/2
  Product4/1 -> Sum5/1
  i_0s/1 -> Product4/2
  Product1/1 -> Sum1/2

== system Consigna5_2_1/Subsystem4/MODULADOR DE TORQUE1/Lazo de Torque ==
  Tm* : Inport
  omega_m : Inport  Port=2
  ids : Inport  Port=3
  Constant : Constant  Value=lambda_m
  Constant1 : Constant  Value=g
  Divide : Product  Inputs=*/
  Integrator : Integrator  InitialCondition=pi/4
  Ld-Lq : Constant  Value=L_d-L_q
  Multiply : Gain  Gain=b_eq
  Multiply1 : Gain  Gain=1/r
  Multiply2 : Gain  Gain=k_l
  Multiply3 : Gain  Gain=1/r
  Multiply5 : Gain  Gain=P_p
  Multiply6 : Gain  Gain=3/2
  Product : Product
  Product1 : Product
  Sin : Trigonometry
  Sum1 : Sum  Inputs=|++
  Sum2 : Sum  Inputs=|+++
  iqs* : Outport
  wires:
  Constant/1 -> Sum1/2
  Ld-Lq/1 -> Product1/2
  omega_m/1 -> Integrator/1, Multiply/1
  Tm*/1 -> Sum2/1
  ids/1 -> Product1/1
  Multiply3/1 -> Product/1
  Product/1 -> Sum2/3
  Multiply6/1 -> Divide/2
  Multiply2/1 -> Multiply3/1
  Integrator/1 -> Multiply1/1
  Multiply1/1 -> Sin/1
  Multiply/1 -> Sum2/2
  Sum2/1 -> Divide/1
  Multiply5/1 -> Multiply6/1
  Divide/1 -> iqs*/1
  Sum1/1 -> Multiply5/1
  Sin/1 -> Multiply2/1
  Constant1/1 -> Product/2
  Product1/1 -> Sum1/1

== system Consigna5_2_1/Subsystem4/MODULADOR DE TORQUE1/Modulador de corriente ==
  I_qs* : Inport
  I_ds* : Inport  Port=2
  I_0s* : Inport  Port=3
  i_qs : Inport  Port=4
  i_ds : Inport  Port=5
  i_0s : Inport  Port=6
  Gain : Gain  Gain=5000*L_q
  Gain1 : Gain  Gain=5000*L_d
  Gain2 : Gain  Gain=5000*L_ls
  Sum : Sum  Inputs=+-
  Sum1 : Sum  Inputs=+-
  Sum2 : Sum  Inputs=+-
  v_qs* : Outport
  v_ds* : Outport  Port=2
  v_0s* : Outport  Port=3
  wires:
  Sum2/1 -> Gain2/1
  Sum1/1 -> Gain1/1
  Sum/1 -> Gain/1
  I_qs*/1 -> Sum/1
  i_qs/1 -> Sum/2
  I_ds*/1 -> Sum1/1
  i_ds/1 -> Sum1/2
  I_0s*/1 -> Sum2/1
  i_0s/1 -> Sum2/2
  Gain/1 -> v_qs*/1
  Gain2/1 -> v_0s*/1
  Gain1/1 -> v_ds*/1

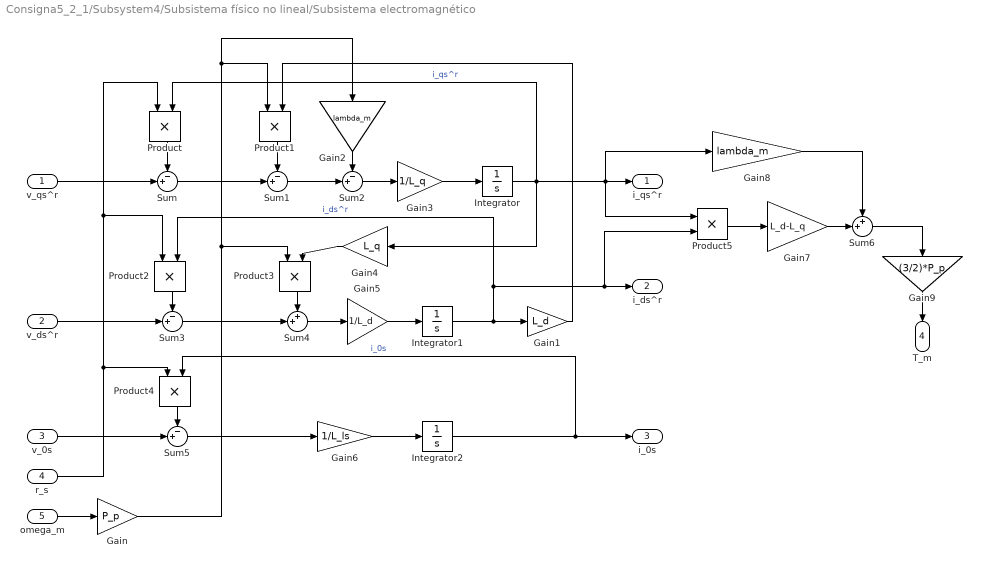
== system Consigna5_2_1/Subsystem4/Subsistema físico no lineal/Subsistema electromagnético ==
  v_qs^r : Inport
  v_ds^r : Inport  Port=2
  v_0s : Inport  Port=3
  r_s : Inport  Port=4
  omega_m : Inport  Port=5
  Gain : Gain  Gain=P_p
  Gain1 : Gain  Gain=L_d
  Gain2 : Gain  Gain=lambda_m
  Gain3 : Gain  Gain=1/L_q
  Gain4 : Gain  Gain=L_q
  Gain5 : Gain  Gain=1/L_d
  Gain6 : Gain  Gain=1/L_ls
  Gain7 : Gain  Gain=L_d-L_q
  Gain8 : Gain  Gain=lambda_m
  Gain9 : Gain  Gain=(3/2)*P_p
  Integrator : Integrator
  Integrator1 : Integrator
  Integrator2 : Integrator
  Product{,1..5} (6 alike) : Product
  Sum{,1..3,5} (5 alike) : Sum  Inputs=-+|
  Sum4 : Sum  Inputs=++|
  Sum6 : Sum  Inputs=++|
  i_qs^r : Outport
  i_ds^r : Outport  Port=2
  i_0s : Outport  Port=3
  T_m : Outport  Port=4
  wires:
  v_qs^r/1 -> Sum/2
  Product/1 -> Sum/1
  Sum/1 -> Sum1/2
  Integrator/1 -> Gain8/1, Product5/1, i_qs^r/1, Product/2, Gain4/1  "i_qs^r"
  omega_m/1 -> Gain/1
  Gain/1 -> Gain2/1, Product1/1, Product3/1
  Integrator1/1 -> Product2/2, Product5/2, i_ds^r/1, Gain1/1  "i_ds^r"
  Gain1/1 -> Product1/2
  Sum1/1 -> Sum2/2
  Sum2/1 -> Gain3/1
  Gain2/1 -> Sum2/1
  Product1/1 -> Sum1/1
  Gain3/1 -> Integrator/1
  Product2/1 -> Sum3/1
  v_ds^r/1 -> Sum3/2
  Sum3/1 -> Sum4/2
  Product3/1 -> Sum4/1
  Gain4/1 -> Product3/2
  Gain5/1 -> Integrator1/1
  Sum4/1 -> Gain5/1
  Integrator2/1 -> Product4/2, i_0s/1  "i_0s"
  r_s/1 -> Product4/1, Product/1, Product2/1
  Product4/1 -> Sum5/1
  v_0s/1 -> Sum5/2
  Sum5/1 -> Gain6/1
  Gain6/1 -> Integrator2/1
  Product5/1 -> Gain7/1
  Gain7/1 -> Sum6/2
  Gain8/1 -> Sum6/1
  Sum6/1 -> Gain9/1
  Gain9/1 -> T_m/1

== system Consigna5_2_1/Subsystem4/Subsistema físico no lineal/Subsistema mecánico completo ==
  T_m : Inport
  T_l : Inport  Port=2
  Gain : Gain  Gain=b_m + b_l / (r^2)
  Gain1 : Gain  Gain=1/r
  Gain2 : Gain  Gain=1/(J_m + J_l / r^2)
  Sum : Sum  Inputs=-+-
  omega_m(0) = 0 : Integrator
  theta_m(0) = 0 : Integrator
  theta_m(t) : Outport
  omega_m(t) : Outport  Port=2
  wires:
  Gain2/1 -> omega_m(0) = 0/1  "domega_m(t)/dt"
  Gain1/1 -> Sum/1
  theta_m(0) = 0/1 -> theta_m(t)/1  "theta_m(t)"
  omega_m(0) = 0/1 -> omega_m(t)/1, Gain/1, theta_m(0) = 0/1  "omega_m(t)"
  Sum/1 -> Gain2/1
  Gain/1 -> Sum/3
  T_l/1 -> Gain1/1
  T_m/1 -> Sum/2

== system Consigna5_2_1/Subsystem4/Subsistema físico no lineal/Subsistema térmico ==
  i_qs^r : Inport
  i_ds^r : Inport  Port=2
  i_0s^r : Inport  Port=3
  Tº_amb : Inport  Port=4
  Constant : Constant  Value=Temp_s_ref
  Constant1 : Constant
  Gain : Gain  Gain=1/C_ts
  Gain1 : Gain  Gain=3/2
  Gain2 : Gain  Gain=1/R_ts_amb
  Gain3 : Gain  Gain=alpha_cu
  Gain4 : Gain  Gain=R_s_40
  Gain5 : Gain  Gain=2
  Integrator : Integrator  InitialCondition=20
  Product : Product
  Square : Math  Operator=square
  Square1 : Math  Operator=square
  Square2 : Math  Operator=square
  Sum : Sum  Inputs=+++
  Sum1 : Sum  Inputs=-|+
  Sum2 : Sum  Inputs=|+-
  Sum3 : Sum  Inputs=|+-
  Sum4 : Sum  Inputs=|++
  r_s : Outport
  T_s : Outport  Port=2
  wires:
  i_qs^r/1 -> Square/1
  i_ds^r/1 -> Square1/1
  i_0s^r/1 -> Square2/1
  Gain/1 -> Integrator/1
  Square/1 -> Sum/1
  Square1/1 -> Sum/2
  Sum/1 -> Product/1
  Product/1 -> Gain1/1
  Tº_amb/1 -> Sum1/1
  Integrator/1 -> T_s/1, Sum3/1, Sum1/2
  Sum1/1 -> Gain2/1
  Gain1/1 -> Sum2/1
  Gain2/1 -> Sum2/2
  Sum2/1 -> Gain/1
  Constant/1 -> Sum3/2
  Sum3/1 -> Gain3/1
  Gain3/1 -> Sum4/1
  Constant1/1 -> Sum4/2
  Sum4/1 -> Gain4/1
  Gain4/1 -> Product/2, r_s/1
  Square2/1 -> Gain5/1
  Gain5/1 -> Sum/3

== system Consigna5_2_1/Subsystem5/MODULADOR DE TORQUE1/Calculo rs ==
  Ts : Inport
  Constant : Constant
  Constant1 : Constant  Value=Temp_s_ref
  Gain : Gain  Gain=alpha_cu
  Gain1 : Gain  Gain=R_s_40
  Sum : Sum  Inputs=|++
  Sum1 : Sum  Inputs=|-+
  r_s : Outport
  wires:
  Constant/1 -> Sum/1
  Gain/1 -> Sum/2
  Ts/1 -> Sum1/2
  Constant1/1 -> Sum1/1
  Sum1/1 -> Gain/1
  Sum/1 -> Gain1/1
  Gain1/1 -> r_s/1

== system Consigna5_2_1/Subsystem5/MODULADOR DE TORQUE1/Desacoples Fisicos ==
  v_qs* : Inport
  v_ds* : Inport  Port=2
  v_0s* : Inport  Port=3
  i_qs : Inport  Port=4
  i_ds : Inport  Port=5
  i_0s : Inport  Port=6
  omega_m : Inport  Port=7
  R_s : Inport  Port=8
  Constant : Constant  Value=lambda_m
  Gain : Gain  Gain=P_p
  Gain1 : Gain  Gain=L_d
  Gain2 : Gain  Gain=L_q*P_p
  Product{,1..4} (5 alike) : Product
  Sum : Sum  Inputs=|++
  Sum1 : Sum  Inputs=|++
  Sum2 : Sum  Inputs=++|
  Sum3 : Sum  Inputs=+-|
  Sum4 : Sum  Inputs=|++
  Sum5 : Sum  Inputs=++|
  v_qs*' : Outport
  v_ds*' : Outport  Port=2
  v_0s*' : Outport  Port=3
  wires:
  Gain/1 -> Product1/2
  Product2/1 -> Sum3/1
  Sum2/1 -> Product1/1
  Sum1/1 -> v_qs*'/1
  i_ds/1 -> Gain1/1, Product2/2
  i_qs/1 -> Gain2/1, Product/2
  v_qs*/1 -> Sum/1
  v_0s*/1 -> Sum5/2
  v_ds*/1 -> Sum4/1
  Sum/1 -> Sum1/1
  R_s/1 -> Product2/1, Product4/1, Product/1
  Sum4/1 -> v_ds*'/1
  Gain2/1 -> Product3/1
  Sum5/1 -> v_0s*'/1
  Product3/1 -> Sum3/2
  omega_m/1 -> Product3/2, Gain/1
  Constant/1 -> Sum2/1
  Product/1 -> Sum/2
  Gain1/1 -> Sum2/2
  Sum3/1 -> Sum4/2
  Product4/1 -> Sum5/1
  i_0s/1 -> Product4/2
  Product1/1 -> Sum1/2

== system Consigna5_2_1/Subsystem5/MODULADOR DE TORQUE1/Lazo de Torque ==
  Tm* : Inport
  omega_m : Inport  Port=2
  ids : Inport  Port=3
  Constant : Constant  Value=lambda_m
  Constant1 : Constant  Value=g
  Divide : Product  Inputs=*/
  Integrator : Integrator  InitialCondition=pi/4
  Ld-Lq : Constant  Value=L_d-L_q
  Multiply : Gain  Gain=b_eq
  Multiply1 : Gain  Gain=1/r
  Multiply2 : Gain  Gain=k_l
  Multiply3 : Gain  Gain=1/r
  Multiply5 : Gain  Gain=P_p
  Multiply6 : Gain  Gain=3/2
  Product : Product
  Product1 : Product
  Sin : Trigonometry
  Sum1 : Sum  Inputs=|++
  Sum2 : Sum  Inputs=|+++
  iqs* : Outport
  wires:
  Constant/1 -> Sum1/2
  Ld-Lq/1 -> Product1/2
  omega_m/1 -> Integrator/1, Multiply/1
  Tm*/1 -> Sum2/1
  ids/1 -> Product1/1
  Multiply3/1 -> Product/1
  Product/1 -> Sum2/3
  Multiply6/1 -> Divide/2
  Multiply2/1 -> Multiply3/1
  Integrator/1 -> Multiply1/1
  Multiply1/1 -> Sin/1
  Multiply/1 -> Sum2/2
  Sum2/1 -> Divide/1
  Multiply5/1 -> Multiply6/1
  Divide/1 -> iqs*/1
  Sum1/1 -> Multiply5/1
  Sin/1 -> Multiply2/1
  Constant1/1 -> Product/2
  Product1/1 -> Sum1/1

== system Consigna5_2_1/Subsystem5/MODULADOR DE TORQUE1/Modulador de corriente ==
  I_qs* : Inport
  I_ds* : Inport  Port=2
  I_0s* : Inport  Port=3
  i_qs : Inport  Port=4
  i_ds : Inport  Port=5
  i_0s : Inport  Port=6
  Gain : Gain  Gain=5000*L_q
  Gain1 : Gain  Gain=5000*L_d
  Gain2 : Gain  Gain=5000*L_ls
  Sum : Sum  Inputs=+-
  Sum1 : Sum  Inputs=+-
  Sum2 : Sum  Inputs=+-
  v_qs* : Outport
  v_ds* : Outport  Port=2
  v_0s* : Outport  Port=3
  wires:
  Sum2/1 -> Gain2/1
  Sum1/1 -> Gain1/1
  Sum/1 -> Gain/1
  I_qs*/1 -> Sum/1
  i_qs/1 -> Sum/2
  I_ds*/1 -> Sum1/1
  i_ds/1 -> Sum1/2
  I_0s*/1 -> Sum2/1
  i_0s/1 -> Sum2/2
  Gain/1 -> v_qs*/1
  Gain2/1 -> v_0s*/1
  Gain1/1 -> v_ds*/1

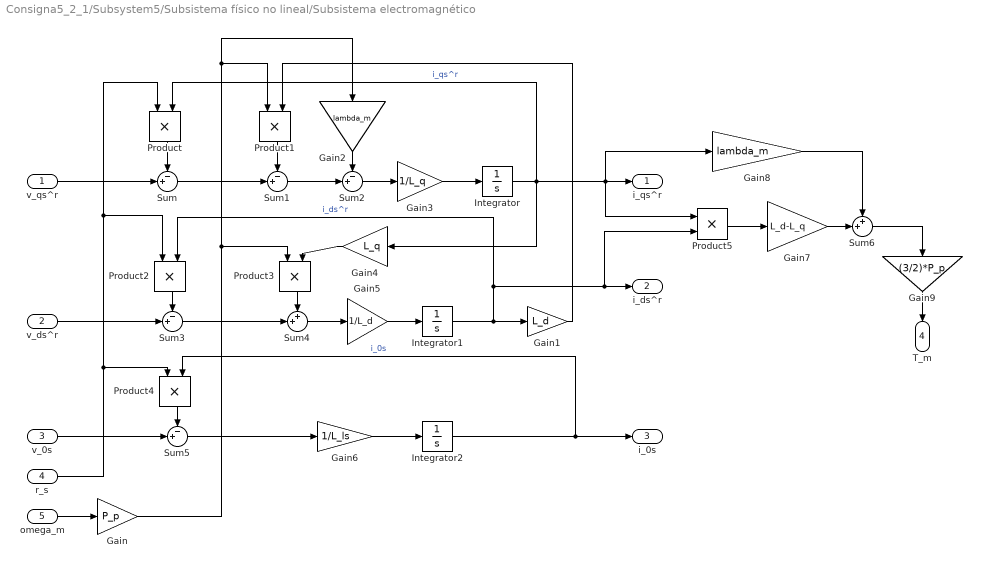
== system Consigna5_2_1/Subsystem5/Subsistema físico no lineal/Subsistema electromagnético ==
  v_qs^r : Inport
  v_ds^r : Inport  Port=2
  v_0s : Inport  Port=3
  r_s : Inport  Port=4
  omega_m : Inport  Port=5
  Gain : Gain  Gain=P_p
  Gain1 : Gain  Gain=L_d
  Gain2 : Gain  Gain=lambda_m
  Gain3 : Gain  Gain=1/L_q
  Gain4 : Gain  Gain=L_q
  Gain5 : Gain  Gain=1/L_d
  Gain6 : Gain  Gain=1/L_ls
  Gain7 : Gain  Gain=L_d-L_q
  Gain8 : Gain  Gain=lambda_m
  Gain9 : Gain  Gain=(3/2)*P_p
  Integrator : Integrator
  Integrator1 : Integrator
  Integrator2 : Integrator
  Product{,1..5} (6 alike) : Product
  Sum{,1..3,5} (5 alike) : Sum  Inputs=-+|
  Sum4 : Sum  Inputs=++|
  Sum6 : Sum  Inputs=++|
  i_qs^r : Outport
  i_ds^r : Outport  Port=2
  i_0s : Outport  Port=3
  T_m : Outport  Port=4
  wires:
  v_qs^r/1 -> Sum/2
  Product/1 -> Sum/1
  Sum/1 -> Sum1/2
  Integrator/1 -> Gain8/1, Product5/1, i_qs^r/1, Product/2, Gain4/1  "i_qs^r"
  omega_m/1 -> Gain/1
  Gain/1 -> Gain2/1, Product1/1, Product3/1
  Integrator1/1 -> Product2/2, Product5/2, i_ds^r/1, Gain1/1  "i_ds^r"
  Gain1/1 -> Product1/2
  Sum1/1 -> Sum2/2
  Sum2/1 -> Gain3/1
  Gain2/1 -> Sum2/1
  Product1/1 -> Sum1/1
  Gain3/1 -> Integrator/1
  Product2/1 -> Sum3/1
  v_ds^r/1 -> Sum3/2
  Sum3/1 -> Sum4/2
  Product3/1 -> Sum4/1
  Gain4/1 -> Product3/2
  Gain5/1 -> Integrator1/1
  Sum4/1 -> Gain5/1
  Integrator2/1 -> Product4/2, i_0s/1  "i_0s"
  r_s/1 -> Product4/1, Product/1, Product2/1
  Product4/1 -> Sum5/1
  v_0s/1 -> Sum5/2
  Sum5/1 -> Gain6/1
  Gain6/1 -> Integrator2/1
  Product5/1 -> Gain7/1
  Gain7/1 -> Sum6/2
  Gain8/1 -> Sum6/1
  Sum6/1 -> Gain9/1
  Gain9/1 -> T_m/1

== system Consigna5_2_1/Subsystem5/Subsistema físico no lineal/Subsistema mecánico completo ==
  T_m : Inport
  T_l : Inport  Port=2
  Gain : Gain  Gain=b_m + b_l / (r^2)
  Gain1 : Gain  Gain=1/r
  Gain2 : Gain  Gain=1/(J_m + J_l / r^2)
  Sum : Sum  Inputs=-+-
  omega_m(0) = 0 : Integrator
  theta_m(0) = 0 : Integrator
  theta_m(t) : Outport
  omega_m(t) : Outport  Port=2
  wires:
  Gain2/1 -> omega_m(0) = 0/1  "domega_m(t)/dt"
  Gain1/1 -> Sum/1
  theta_m(0) = 0/1 -> theta_m(t)/1  "theta_m(t)"
  omega_m(0) = 0/1 -> omega_m(t)/1, Gain/1, theta_m(0) = 0/1  "omega_m(t)"
  Sum/1 -> Gain2/1
  Gain/1 -> Sum/3
  T_l/1 -> Gain1/1
  T_m/1 -> Sum/2

== system Consigna5_2_1/Subsystem5/Subsistema físico no lineal/Subsistema térmico ==
  i_qs^r : Inport
  i_ds^r : Inport  Port=2
  i_0s^r : Inport  Port=3
  Tº_amb : Inport  Port=4
  Constant : Constant  Value=Temp_s_ref
  Constant1 : Constant
  Gain : Gain  Gain=1/C_ts
  Gain1 : Gain  Gain=3/2
  Gain2 : Gain  Gain=1/R_ts_amb
  Gain3 : Gain  Gain=alpha_cu
  Gain4 : Gain  Gain=R_s_40
  Gain5 : Gain  Gain=2
  Integrator : Integrator  InitialCondition=20
  Product : Product
  Square : Math  Operator=square
  Square1 : Math  Operator=square
  Square2 : Math  Operator=square
  Sum : Sum  Inputs=+++
  Sum1 : Sum  Inputs=-|+
  Sum2 : Sum  Inputs=|+-
  Sum3 : Sum  Inputs=|+-
  Sum4 : Sum  Inputs=|++
  r_s : Outport
  T_s : Outport  Port=2
  wires:
  i_qs^r/1 -> Square/1
  i_ds^r/1 -> Square1/1
  i_0s^r/1 -> Square2/1
  Gain/1 -> Integrator/1
  Square/1 -> Sum/1
  Square1/1 -> Sum/2
  Sum/1 -> Product/1
  Product/1 -> Gain1/1
  Tº_amb/1 -> Sum1/1
  Integrator/1 -> T_s/1, Sum3/1, Sum1/2
  Sum1/1 -> Gain2/1
  Gain1/1 -> Sum2/1
  Gain2/1 -> Sum2/2
  Sum2/1 -> Gain/1
  Constant/1 -> Sum3/2
  Sum3/1 -> Gain3/1
  Gain3/1 -> Sum4/1
  Constant1/1 -> Sum4/2
  Sum4/1 -> Gain4/1
  Gain4/1 -> Product/2, r_s/1
  Square2/1 -> Gain5/1
  Gain5/1 -> Sum/3

== system Consigna5_2_1/Subsystem6/MODULADOR DE TORQUE1/Calculo rs ==
  Ts : Inport
  Constant : Constant
  Constant1 : Constant  Value=Temp_s_ref
  Gain : Gain  Gain=alpha_cu
  Gain1 : Gain  Gain=R_s_40
  Sum : Sum  Inputs=|++
  Sum1 : Sum  Inputs=|-+
  r_s : Outport
  wires:
  Constant/1 -> Sum/1
  Gain/1 -> Sum/2
  Ts/1 -> Sum1/2
  Constant1/1 -> Sum1/1
  Sum1/1 -> Gain/1
  Sum/1 -> Gain1/1
  Gain1/1 -> r_s/1

== system Consigna5_2_1/Subsystem6/MODULADOR DE TORQUE1/Desacoples Fisicos ==
  v_qs* : Inport
  v_ds* : Inport  Port=2
  v_0s* : Inport  Port=3
  i_qs : Inport  Port=4
  i_ds : Inport  Port=5
  i_0s : Inport  Port=6
  omega_m : Inport  Port=7
  R_s : Inport  Port=8
  Constant : Constant  Value=lambda_m
  Gain : Gain  Gain=P_p
  Gain1 : Gain  Gain=L_d
  Gain2 : Gain  Gain=L_q*P_p
  Product{,1..4} (5 alike) : Product
  Sum : Sum  Inputs=|++
  Sum1 : Sum  Inputs=|++
  Sum2 : Sum  Inputs=++|
  Sum3 : Sum  Inputs=+-|
  Sum4 : Sum  Inputs=|++
  Sum5 : Sum  Inputs=++|
  v_qs*' : Outport
  v_ds*' : Outport  Port=2
  v_0s*' : Outport  Port=3
  wires:
  Gain/1 -> Product1/2
  Product2/1 -> Sum3/1
  Sum2/1 -> Product1/1
  Sum1/1 -> v_qs*'/1
  i_ds/1 -> Gain1/1, Product2/2
  i_qs/1 -> Gain2/1, Product/2
  v_qs*/1 -> Sum/1
  v_0s*/1 -> Sum5/2
  v_ds*/1 -> Sum4/1
  Sum/1 -> Sum1/1
  R_s/1 -> Product2/1, Product4/1, Product/1
  Sum4/1 -> v_ds*'/1
  Gain2/1 -> Product3/1
  Sum5/1 -> v_0s*'/1
  Product3/1 -> Sum3/2
  omega_m/1 -> Product3/2, Gain/1
  Constant/1 -> Sum2/1
  Product/1 -> Sum/2
  Gain1/1 -> Sum2/2
  Sum3/1 -> Sum4/2
  Product4/1 -> Sum5/1
  i_0s/1 -> Product4/2
  Product1/1 -> Sum1/2

== system Consigna5_2_1/Subsystem6/MODULADOR DE TORQUE1/Lazo de Torque ==
  Tm* : Inport
  omega_m : Inport  Port=2
  ids : Inport  Port=3
  Constant : Constant  Value=lambda_m
  Constant1 : Constant  Value=g
  Divide : Product  Inputs=*/
  Integrator : Integrator  InitialCondition=pi/4
  Ld-Lq : Constant  Value=L_d-L_q
  Multiply : Gain  Gain=b_eq
  Multiply1 : Gain  Gain=1/r
  Multiply2 : Gain  Gain=k_l
  Multiply3 : Gain  Gain=1/r
  Multiply5 : Gain  Gain=P_p
  Multiply6 : Gain  Gain=3/2
  Product : Product
  Product1 : Product
  Sin : Trigonometry
  Sum1 : Sum  Inputs=|++
  Sum2 : Sum  Inputs=|+++
  iqs* : Outport
  wires:
  Constant/1 -> Sum1/2
  Ld-Lq/1 -> Product1/2
  omega_m/1 -> Integrator/1, Multiply/1
  Tm*/1 -> Sum2/1
  ids/1 -> Product1/1
  Multiply3/1 -> Product/1
  Product/1 -> Sum2/3
  Multiply6/1 -> Divide/2
  Multiply2/1 -> Multiply3/1
  Integrator/1 -> Multiply1/1
  Multiply1/1 -> Sin/1
  Multiply/1 -> Sum2/2
  Sum2/1 -> Divide/1
  Multiply5/1 -> Multiply6/1
  Divide/1 -> iqs*/1
  Sum1/1 -> Multiply5/1
  Sin/1 -> Multiply2/1
  Constant1/1 -> Product/2
  Product1/1 -> Sum1/1

== system Consigna5_2_1/Subsystem6/MODULADOR DE TORQUE1/Modulador de corriente ==
  I_qs* : Inport
  I_ds* : Inport  Port=2
  I_0s* : Inport  Port=3
  i_qs : Inport  Port=4
  i_ds : Inport  Port=5
  i_0s : Inport  Port=6
  Gain : Gain  Gain=5000*L_q
  Gain1 : Gain  Gain=5000*L_d
  Gain2 : Gain  Gain=5000*L_ls
  Sum : Sum  Inputs=+-
  Sum1 : Sum  Inputs=+-
  Sum2 : Sum  Inputs=+-
  v_qs* : Outport
  v_ds* : Outport  Port=2
  v_0s* : Outport  Port=3
  wires:
  Sum2/1 -> Gain2/1
  Sum1/1 -> Gain1/1
  Sum/1 -> Gain/1
  I_qs*/1 -> Sum/1
  i_qs/1 -> Sum/2
  I_ds*/1 -> Sum1/1
  i_ds/1 -> Sum1/2
  I_0s*/1 -> Sum2/1
  i_0s/1 -> Sum2/2
  Gain/1 -> v_qs*/1
  Gain2/1 -> v_0s*/1
  Gain1/1 -> v_ds*/1

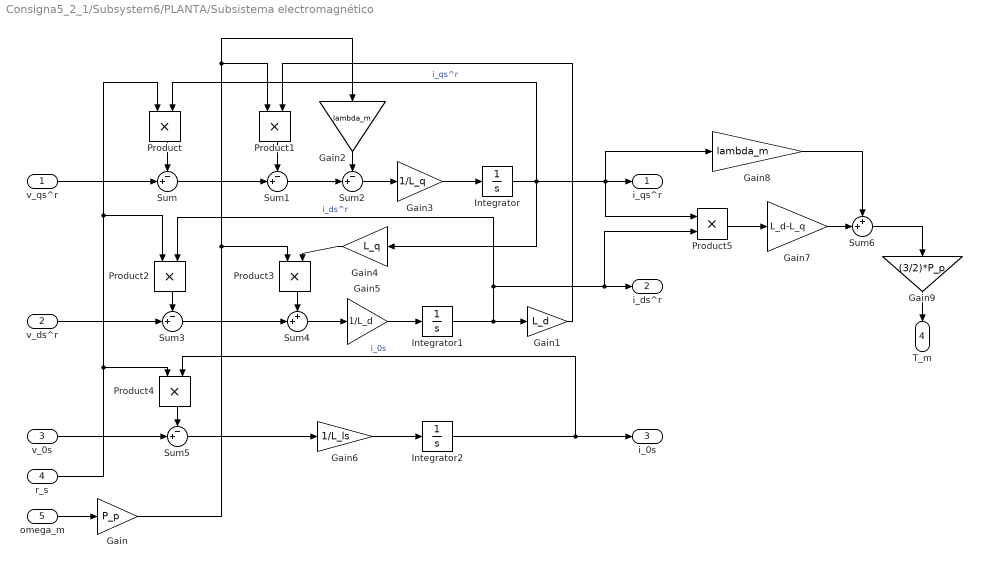
== system Consigna5_2_1/Subsystem6/PLANTA/Subsistema electromagnético ==
  v_qs^r : Inport
  v_ds^r : Inport  Port=2
  v_0s : Inport  Port=3
  r_s : Inport  Port=4
  omega_m : Inport  Port=5
  Gain : Gain  Gain=P_p
  Gain1 : Gain  Gain=L_d
  Gain2 : Gain  Gain=lambda_m
  Gain3 : Gain  Gain=1/L_q
  Gain4 : Gain  Gain=L_q
  Gain5 : Gain  Gain=1/L_d
  Gain6 : Gain  Gain=1/L_ls
  Gain7 : Gain  Gain=L_d-L_q
  Gain8 : Gain  Gain=lambda_m
  Gain9 : Gain  Gain=(3/2)*P_p
  Integrator : Integrator
  Integrator1 : Integrator
  Integrator2 : Integrator
  Product{,1..5} (6 alike) : Product
  Sum{,1..3,5} (5 alike) : Sum  Inputs=-+|
  Sum4 : Sum  Inputs=++|
  Sum6 : Sum  Inputs=++|
  i_qs^r : Outport
  i_ds^r : Outport  Port=2
  i_0s : Outport  Port=3
  T_m : Outport  Port=4
  wires:
  v_qs^r/1 -> Sum/2
  Product/1 -> Sum/1
  Sum/1 -> Sum1/2
  Integrator/1 -> Gain8/1, Product5/1, i_qs^r/1, Product/2, Gain4/1  "i_qs^r"
  omega_m/1 -> Gain/1
  Gain/1 -> Gain2/1, Product1/1, Product3/1
  Integrator1/1 -> Product2/2, Product5/2, i_ds^r/1, Gain1/1  "i_ds^r"
  Gain1/1 -> Product1/2
  Sum1/1 -> Sum2/2
  Sum2/1 -> Gain3/1
  Gain2/1 -> Sum2/1
  Product1/1 -> Sum1/1
  Gain3/1 -> Integrator/1
  Product2/1 -> Sum3/1
  v_ds^r/1 -> Sum3/2
  Sum3/1 -> Sum4/2
  Product3/1 -> Sum4/1
  Gain4/1 -> Product3/2
  Gain5/1 -> Integrator1/1
  Sum4/1 -> Gain5/1
  Integrator2/1 -> Product4/2, i_0s/1  "i_0s"
  r_s/1 -> Product4/1, Product/1, Product2/1
  Product4/1 -> Sum5/1
  v_0s/1 -> Sum5/2
  Sum5/1 -> Gain6/1
  Gain6/1 -> Integrator2/1
  Product5/1 -> Gain7/1
  Gain7/1 -> Sum6/2
  Gain8/1 -> Sum6/1
  Sum6/1 -> Gain9/1
  Gain9/1 -> T_m/1

== system Consigna5_2_1/Subsystem6/PLANTA/Subsistema mecánico completo ==
  T_m : Inport
  T_l : Inport  Port=2
  Gain : Gain  Gain=b_m + b_l / (r^2)
  Gain1 : Gain  Gain=1/r
  Gain2 : Gain  Gain=1/(J_m + J_l / r^2)
  Sum : Sum  Inputs=-+-
  omega_m(0) = 0 : Integrator
  theta_m(0) = 0 : Integrator
  theta_m(t) : Outport
  omega_m(t) : Outport  Port=2
  wires:
  Gain2/1 -> omega_m(0) = 0/1  "domega_m(t)/dt"
  Gain1/1 -> Sum/1
  theta_m(0) = 0/1 -> theta_m(t)/1  "theta_m(t)"
  omega_m(0) = 0/1 -> omega_m(t)/1, Gain/1, theta_m(0) = 0/1  "omega_m(t)"
  Sum/1 -> Gain2/1
  Gain/1 -> Sum/3
  T_l/1 -> Gain1/1
  T_m/1 -> Sum/2
